simulink model "part1"  (R2018b)
settings: Solver=FixedStepAuto  StartTime=0.0  StopTime=10.0  FixedStep=1e-3  RelTol=1e-3  EnableMultiTasking=on
undefined symbols (not defined in the file): D10, D12, D2, D5, D9, PTA2, PTB9, PTC4, PTD0, PTD3
libraries: frdmk64flib x5
settings Model: ExtModeTrigDuration=5  Creator=Siddharth  LastModifiedBy=Buggs
settings OptimizationCC: PassReuseOutputArgsAs=Individual arguments  MaxStackSize=64
settings DebuggingCC: ParameterTunabilityLossMsg=error
settings HardwareCC: ProdBitPerPointer=32  ProdBitPerSizeT=32  ProdBitPerPtrDiffT=32  ProdLargestAtomicInteger=Long  ProdLargestAtomicFloat=Double  ProdWordSize=32  ProdHWDeviceType=ARM Compatible->ARM Cortex
settings SFSimCC: SimUseLocalCustomCode=off  MATLABDynamicMemAlloc=off
settings RTWCC: SystemTargetFile=ert.tlc  HardwareBoard=NXP FRDM-K64F  TLCOptions="-aInlineSetEventsForThisBaseRateFcn=TLC_FALSE -aSuppressMultiTaskScheduler=TLC_FALSE  -aRateBasedStepFcn=0"  TemplateMakefile=ert_default_tmf  GenerateReport=on  RTWUseLocalCustomCode=off  Toolchain=GNU Tools for ARM Embedded Processors  IncludeHyperlinkInReport=on  LaunchReport=on  GenerateTraceInfo=on  GenerateTraceReport=on  GenerateTraceReportSl=on  GenerateTraceReportSf=on  GenerateTraceReportEml=on
settings CodeAppCC: ForceParamTrailComments=on  IgnoreCustomStorageClasses=off  OperatorAnnotations=on  SimulinkDataObjDesc=on  SFDataObjDesc=on  InsertBlockDesc=on

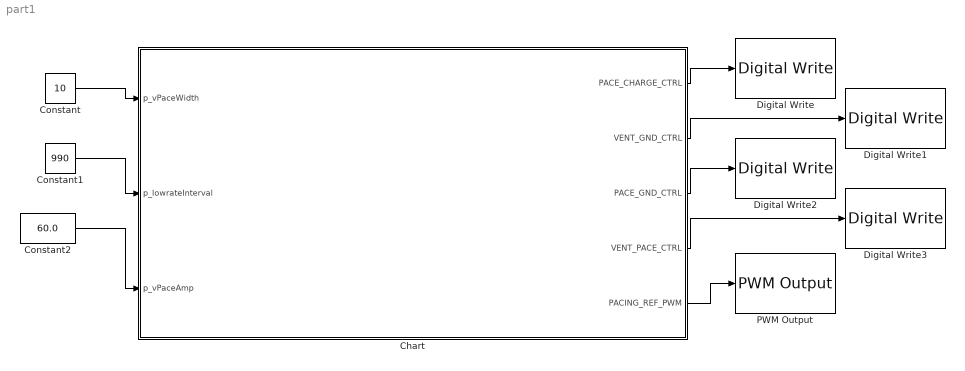
== system part1 ==
  Chart : Stateflow chart  TreatAsAtomicUnit=on
  Constant : Constant  Value=10  OutDataTypeStr=int16
  Constant1 : Constant  Value=990  OutDataTypeStr=int16
  Constant2 : Constant  Value=60.0  OutDataTypeStr=double
  Digital Write : frdmk64flib/Digital Write  Whichpin=PTB9 (D2)
      settings: SourceProductName=Simulink Coder Support Package for NXP FRDM-K64F Board
  Digital Write1 : frdmk64flib/Digital Write  Whichpin=PTD3 (D12)
      settings: SourceProductName=Simulink Coder Support Package for NXP FRDM-K64F Board
  Digital Write2 : frdmk64flib/Digital Write  Whichpin=PTD0 (D10)
      settings: SourceProductName=Simulink Coder Support Package for NXP FRDM-K64F Board
  Digital Write3 : frdmk64flib/Digital Write  Whichpin=PTC4 (D9)
      settings: SourceProductName=Simulink Coder Support Package for NXP FRDM-K64F Board
  PWM Output : frdmk64flib/PWM Output  Whichpin=PTA2 (D5)  InitialFrequency=1000  InitialDutyCycle=0
      settings: SourceProductName=Simulink Coder Support Package for NXP FRDM-K64F Board
  wires:
  Chart/5(PACING_REF_PWM) -> PWM Output/1
  Chart/2(VENT_GND_CTRL) -> Digital Write1/1
  Chart/4(VENT_PACE_CTRL) -> Digital Write3/1
  Constant/1 -> Chart/1(p_vPaceWidth)
  Constant2/1 -> Chart/3(p_vPaceAmp)
  Constant1/1 -> Chart/2(p_lowrateInterval)
  Chart/3(PACE_GND_CTRL) -> Digital Write2/1
  Chart/1(PACE_CHARGE_CTRL) -> Digital Write/1

== stateflow chart part1/Chart ==
  state CHARGE_BLOCK
    entry:
    PACE_CHARGE_CTRL=false;
    VENT_PACE_CTRL=true;
    VENT_GND_CTRL=false;
  state DISCHARGE_CHARGE
    entry:
    PACING_REF_PWM=p_vPaceAmp;
    PACE_CHARGE_CTRL=true;
    VENT_PACE_CTRL=false;
    VENT_GND_CTRL=true;
    PACE_GND_CTRL=true;
  (default) -> DISCHARGE_CHARGE
  DISCHARGE_CHARGE -> CHARGE_BLOCK : after(p_lowrateInterval,msec)
  CHARGE_BLOCK -> DISCHARGE_CHARGE : after(p_vPaceWidth,msec)
  data: p_vPaceWidth input int16; p_lowrateInterval input int16; PACE_CHARGE_CTRL output boolean; VENT_GND_CTRL output boolean; PACE_GND_CTRL output boolean; VENT_PACE_CTRL output boolean; PACING_REF_PWM output double; p_vPaceAmp input double
